simulink model "tanks1"  (R2023a)
settings: Solver=VariableStepAuto  StartTime=0.0  StopTime=60  RelTol=1e-3
values from neighbouring files (symbols this model uses):
  a0 = pi * (d0 / 2)^2    (= 1.55528471307e-05)    [calculate_matrix.m]    (also in equilibrum_h.m; param_G3.m)
  A0 = pi * (Di / 2)^2    (= 0.00155179165474)    [calculate_matrix.m]    (also in equilibrum_h.m; param_G3.m)
  A1 = pi * (Di / 2)^2    (= 0.00155179165474)    [calculate_matrix.m]    (also in equilibrum_h.m; param_G3.m)
  a1 = pi * (d1 / 2)^2    (= 2.42471809941e-05)    [calculate_matrix.m]    (also in equilibrum_h.m; param_G3.m)
  a2 = pi * (d0 / 2)^2    (= 1.55528471307e-05)    [calculate_matrix.m]    (also in equilibrum_h.m; param_G3.m)
  A2 = pi * (Di / 2)^2    (= 0.00155179165474)    [calculate_matrix.m]    (also in equilibrum_h.m; param_G3.m)
  A3 = pi * (Di / 2)^2    (= 0.00155179165474)    [calculate_matrix.m]    (also in equilibrum_h.m; param_G3.m)
  a3 = pi * (d1 / 2)^2    (= 2.42471809941e-05)    [calculate_matrix.m]    (also in equilibrum_h.m; param_G3.m)
  g = 9.8    [calculate_matrix.m]    (also in equilibrum_h.m; param_G3.m = 9.81)
  gamma = 0.61    [calculate_matrix.m]    (also in equilibrum_h.m; param_G3.m)
  k0 = 3.9e-6    (= 3.9e-06)    [calculate_matrix.m]    (also in equilibrum_h.m; param_G3.m)
  k1 = 4.15e-6    (= 4.15e-06)    [calculate_matrix.m]    (also in equilibrum_h.m; param_G3.m)
  v1 = 9.5    [calculate_matrix.m]    (also in equilibrum_h.m)
undefined symbols (not defined in the file or in its folder): v0
settings Model: Creator=User  LastModifiedBy=User

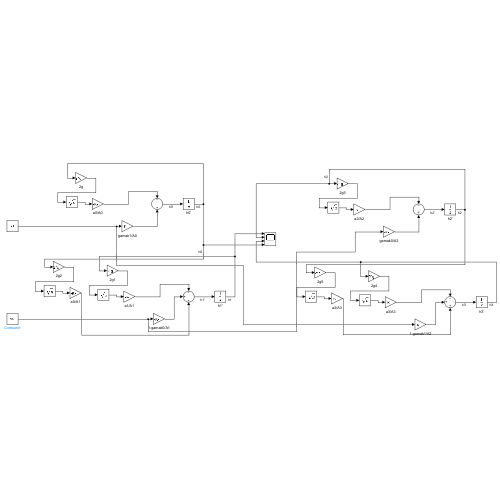
[thumbnail: Simulink's stored preview of the top-level diagram]
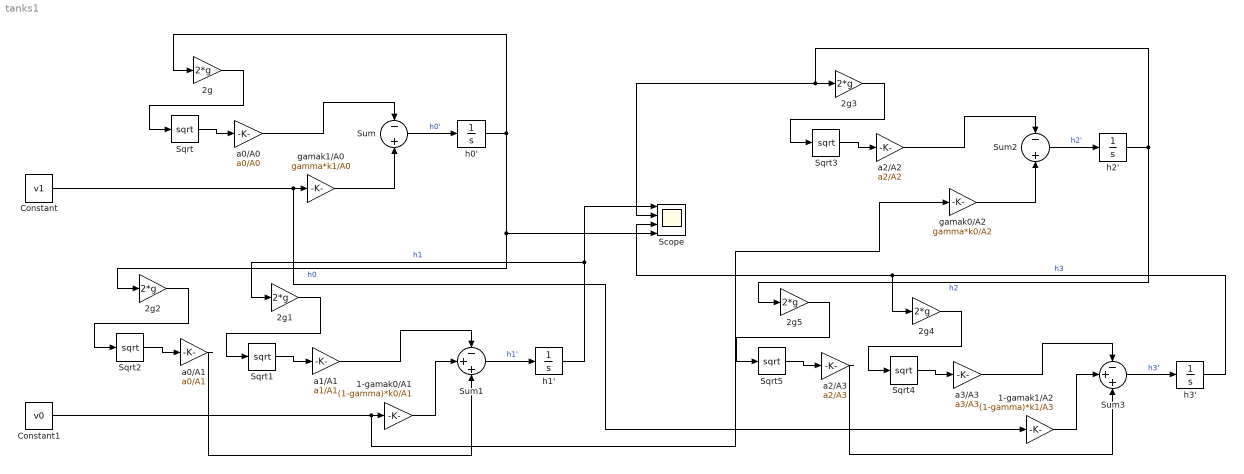
== system tanks1 ==
  1-gamak0/A1 : Gain  Gain=(1-gamma)*k0/A1
  1-gamak1/A2 : Gain  Gain=(1-gamma)*k1/A3
  2g{,1..5} (6 alike) : Gain  Gain=2*g
  Constant : Constant  Value=v1
  Constant1 : Constant  Value=v0
  Scope : Scope  NumInputPorts=4
  Sqrt{,1..5} (6 alike) : Sqrt
  Sum : Sum  Inputs=-+
  Sum1 : Sum  Inputs=-++
  Sum2 : Sum  Inputs=-+
  Sum3 : Sum  Inputs=-++
  a0/A0 : Gain  Gain=a0/A0
  a0/A1 : Gain  Gain=a0/A1
  a1/A1 : Gain  Gain=a1/A1
  a2/A2 : Gain  Gain=a2/A2
  a2/A3 : Gain  Gain=a2/A3
  a3/A3 : Gain  Gain=a3/A3
  gamak0/A2 : Gain  Gain=gamma*k0/A2
  gamak1/A0 : Gain  Gain=gamma*k1/A0
  h0' : Integrator
  h1' : Integrator
  h2' : Integrator
  h3' : Integrator
  wires:
  h0'/1 -> 2g/1, Scope/4, 2g2/1  "h0"
  2g/1 -> Sqrt/1
  Sqrt/1 -> a0/A0/1
  gamak1/A0/1 -> Sum/2
  a0/A0/1 -> Sum/1
  Sum/1 -> h0'/1  "h0'"
  1-gamak0/A1/1 -> Sum1/2
  2g1/1 -> Sqrt1/1
  h1'/1 -> Scope/1, 2g1/1  "h1"
  Sqrt1/1 -> a1/A1/1
  a1/A1/1 -> Sum1/1
  Sum1/1 -> h1'/1  "h1'"
  2g2/1 -> Sqrt2/1
  Sqrt2/1 -> a0/A1/1
  a0/A1/1 -> Sum1/3
  a2/A3/1 -> Sum3/3
  Sum3/1 -> h3'/1  "h3'"
  a3/A3/1 -> Sum3/1
  Constant/1 -> 1-gamak1/A2/1, gamak1/A0/1
  2g4/1 -> Sqrt4/1
  h3'/1 -> Scope/3, 2g4/1  "h3"
  1-gamak1/A2/1 -> Sum3/2
  Sum2/1 -> h2'/1  "h2'"
  Sqrt5/1 -> a2/A3/1
  gamak0/A2/1 -> Sum2/2
  2g3/1 -> Sqrt3/1
  h2'/1 -> Scope/2, 2g3/1, 2g5/1  "h2"
  Sqrt4/1 -> a3/A3/1
  2g5/1 -> Sqrt5/1
  Sqrt3/1 -> a2/A2/1
  Constant1/1 -> gamak0/A2/1, 1-gamak0/A1/1
  a2/A2/1 -> Sum2/1
